simulink model "PLL"  (R2017b)
settings: Solver=VariableStepAuto  StartTime=0.0  StopTime=1  MaxStep=1e-4  RelTol=1e-3  EnableMultiTasking=on
values from neighbouring files (symbols this model uses):
  f = 50    [controlhinf.m]    (also in controlhinf2.m; modelCfg.m; psd_score.m = (1/avgT_samp)/n*(0:floor((n-1)/2)))
settings Model: Creator=jelena  LastModifiedBy=cmpoonsvr
settings SolverCC: AutoInsertRateTranBlk=on
settings DataIOCC: SaveOutput=off  SaveTime=off
settings OptimizationCC: LifeSpan=inf
settings DebuggingCC: SFUnexpectedBacktrackingDiag=warning  SFNoUnconditionalDefaultTransitionDiag=warning  SFExecutionAtInitializationDiag=none
settings CodeAppCC: StateflowObjectComments=on
settings GRTTargetCC: TargetLangStandard=C89/C90 (ANSI)  GeneratePreprocessorConditionals=Disable all
settings ConfigComp: CovMetricSettings=dw  CovHtmlReporting=on  CovSaveCumulativeToWorkspaceVar=on  CovSaveSingleToWorkspaceVar=on  CovExternalEMLEnable=off

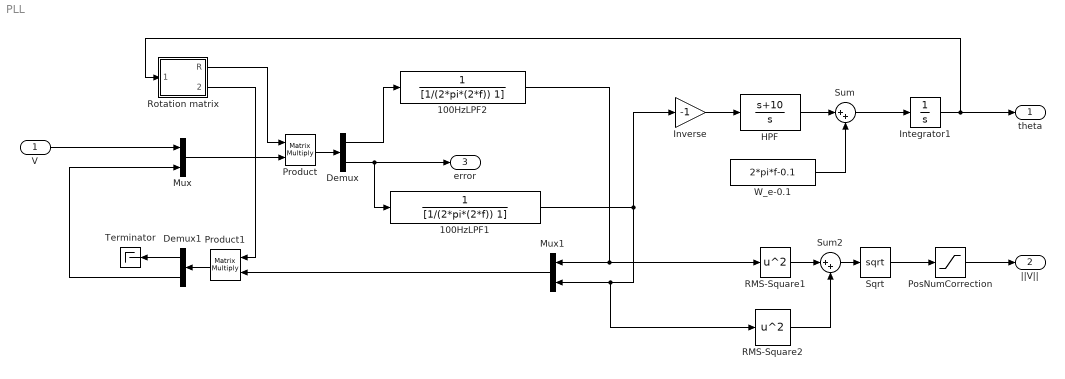
== system PLL ==
  V : Inport  OutDataTypeStr=double  PortDimensions=1  SampleTime=0
  100HzLPF1 : TransferFcn  Denominator=[1/(2*pi*(2*f)) 1]
  100HzLPF2 : TransferFcn  Denominator=[1/(2*pi*(2*f)) 1]
  Demux : Demux  Outputs=2
  Demux1 : Demux  Outputs=2
  HPF : TransferFcn  Numerator=[1 10]  Denominator=[1 0]
  Integrator1 : Integrator  InitialCondition=-pi/2  WrapState=on
  Inverse : Gain  Gain=-1
  Mux : Mux  Inputs=2
  Mux1 : Mux  Inputs=2
  PosNumCorrection : Saturate  UpperLimit=inf  LowerLimit=0.01
  Product : Product  Multiplication=Matrix(*)
  Product1 : Product  Multiplication=Matrix(*)
  RMS-Square1 : Math  Operator=square  SaturateOnIntegerOverflow=on
  RMS-Square2 : Math  Operator=square  SaturateOnIntegerOverflow=on
  Rotation matrix : Subsystem
  Sqrt : Sqrt  SaturateOnIntegerOverflow=on
  Sum : Sum  Inputs=|++
  Sum2 : Sum  Inputs=|++
  Terminator : Terminator
  W_e-0.1 : Constant  Value=2*pi*f-0.1
  theta : Outport  OutDataTypeStr=double  PortDimensions=1  SampleTime=0
  ||V|| : Outport  Port=2  OutDataTypeStr=double  PortDimensions=1  SampleTime=0
  error : Outport  Port=3  OutDataTypeStr=double  PortDimensions=1  SampleTime=0
  wires:
  Mux1/1 -> Product1/2
  Rotation matrix/1(R) -> Product/1
  Product1/1 -> Demux1/1
  Mux/1 -> Product/2
  Demux1/2 -> Mux/2
  100HzLPF1/1 -> Inverse/1, RMS-Square2/1, Mux1/2
  Sum/1 -> Integrator1/1
  HPF/1 -> Sum/1
  Sum2/1 -> Sqrt/1
  RMS-Square1/1 -> Sum2/1
  RMS-Square2/1 -> Sum2/2
  Inverse/1 -> HPF/1
  100HzLPF2/1 -> Mux1/1, RMS-Square1/1
  Demux/1 -> 100HzLPF2/1
  Rotation matrix/2(Rneg) -> Product1/1
  Demux/2 -> 100HzLPF1/1, error/1
  W_e-0.1/1 -> Sum/2
  V/1 -> Mux/1
  Integrator1/1 -> Rotation matrix/1(theta), theta/1
  Product/1 -> Demux/1
  Sqrt/1 -> PosNumCorrection/1
  PosNumCorrection/1 -> ||V||/1
  Demux1/1 -> Terminator/1

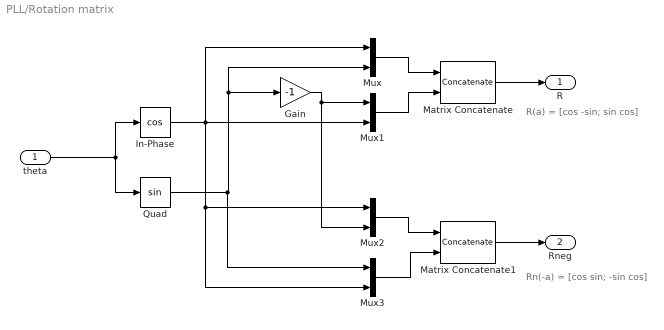
== system PLL/Rotation matrix ==
  note: R(a) = [cos -sin;
      | 	 sin cos]
  note: Rn(-a) = [cos sin;
      | 	 -sin cos]
  theta : Inport
  Gain : Gain  Gain=-1
  In-Phase : Trigonometry  Operator=cos
  Matrix Concatenate : Concatenate  Mode=Multidimensional array  ConcatenateDimension=2
  Matrix Concatenate1 : Concatenate  Mode=Multidimensional array  ConcatenateDimension=2
  Mux{,1..3} (4 alike) : Mux  Inputs=2
  Quad : Trigonometry
  R : Outport
  Rneg : Outport  Port=2
  wires:
  Matrix Concatenate1/1 -> Rneg/1
  Mux3/1 -> Matrix Concatenate1/2
  Mux2/1 -> Matrix Concatenate1/1
  Quad/1 -> Mux/2, Gain/1, Mux3/1
  Gain/1 -> Mux1/1, Mux2/2
  Mux1/1 -> Matrix Concatenate/2
  Mux/1 -> Matrix Concatenate/1
  Matrix Concatenate/1 -> R/1
  In-Phase/1 -> Mux/1, Mux1/2, Mux3/2, Mux2/1
  theta/1 -> Quad/1, In-Phase/1
